simulink model "risk"  (R2025b)
settings: Solver=VariableStepAuto  StartTime=0.0  StopTime=60.0  RelTol=1e-3
libraries: SignalEditorBlockLib x1
settings Model: Creator=hyper  LastModifiedBy=hyper

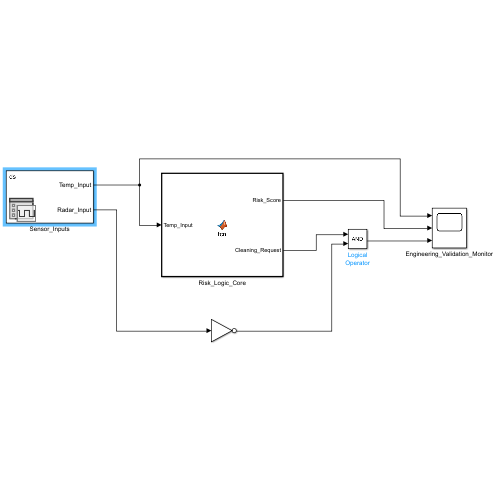
[thumbnail: Simulink's stored preview of the top-level diagram]
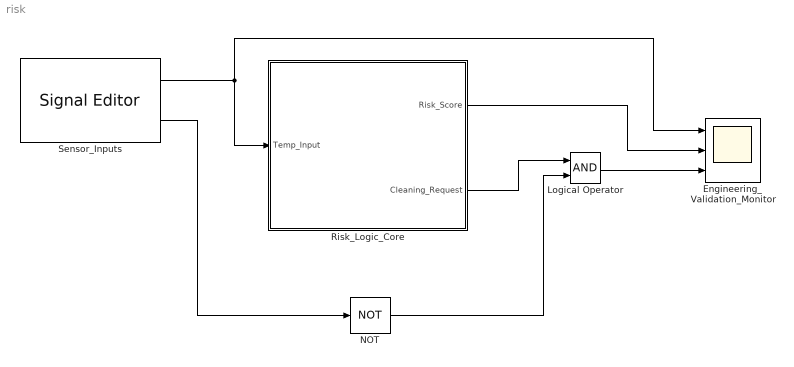
== system risk ==
  Engineering_Validation_Monitor : Scope  NumInputPorts=3
      settings: ActiveDisplayYMinimum=1.8420580247688516  ActiveDisplayYMaximum=63.272533143125166
  Logical Operator : Logic  AllPortsSameDT=off  OutDataTypeStr=boolean
  NOT : Logic  Operator=NOT  IconShape=distinctive  AllPortsSameDT=off  OutDataTypeStr=boolean
  Risk_Logic_Core : MATLAB Function  TreatAsAtomicUnit=on
  Sensor_Inputs : SignalEditorBlockLib/Signal Editor  FileName=patent_data.mat  ActiveScenario=ds  ActiveSignal=Temp_Input  IsBus=off  OutputBusObjectStr=Bus: BusObject  SampleTime=0  ZeroCross=off  OutputAfterFinalValue=Setting to zero  Unit=inherit  PreserveSignalName=on  ApplySigPropsToAllScenarios=on  ApplySigPropsToAllSignals=off  SignalPropertySource=Dialog parameters
  wires:
  Sensor_Inputs/1 -> Risk_Logic_Core/1(Temp_Input), Engineering_Validation_Monitor/1
  Risk_Logic_Core/2(Cleaning_Request) -> Logical Operator/1
  Sensor_Inputs/2 -> NOT/1
  NOT/1 -> Logical Operator/2
  Risk_Logic_Core/1(Risk_Score) -> Engineering_Validation_Monitor/2
  Logical Operator/1 -> Engineering_Validation_Monitor/3

== matlab function risk/Risk_Logic_Core ==
  data: Temp_Input input; Risk_Score output; Cleaning_Request output
function [Risk_Score, Cleaning_Request] = fcn(Temp_Input)
    % PATENT CLAIM 18.b: Risk Calculation Logic
    
    % 1. Define Thresholds
    Fever_Limit = 37.8; 
    Risk_Trigger = 45;  % Score needed to request cleaning

    % 2. Calculate Weights
    w_t = 0;
    if Temp_Input > Fever_Limit
        w_t = 50; % High weight for Fever
    else
        w_t = 0;  % No fever, low risk
    end
    
    % 3. Compute Score
    % (We use a simplified formula for this test: Risk = Fever_Weight)
    Risk_Score = w_t;
    
    % 4. Generate Cleaning Request
    if Risk_Score >= Risk_Trigger
        Cleaning_Request = 1; % TRUE: System wants to clean
    else
        Cleaning_Request = 0; % FALSE: System stays idle
    end
end
